simulink library "Control_FuelCell1Motor"  (R2026a)
settings: Solver=VariableStepAuto
undefined symbols (not defined in the file or in its folder): Coefficient, Control
libraries: simulink x4, Damper_Control_Axle2 x2, sl_discontinuities x2, Driveline_Control_Axle2_None x1, slpidlib x1, Spring_Control_Axle2 x1, Steer_Control_Axle2 x1
Description:
  | Component of Simscape Vehicle Templates Library
  | 
  | Copyright 2018-2026 The MathWorks, Inc.
settings Model: Creator=smiller  LastModifiedBy=smiller

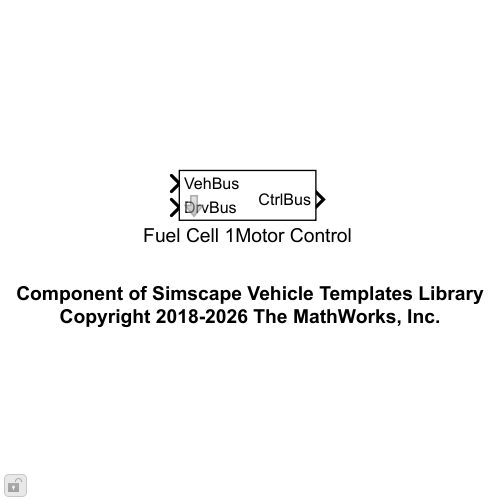
[thumbnail: Simulink's stored preview of the top-level diagram]
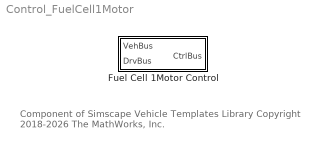
== system Control_FuelCell1Motor ==
  note: Component of Simscape Vehicle Templates Library
      | Copyright 2018-2026 The MathWorks, Inc.
  Fuel Cell 1Motor Control : Subsystem  mask(Control of Fuel Cell Powertrain){ControlFuelCell=Control.FuelCell1Motor, popup_damper_control_A1=Coefficient, popup_damper_control_A2=Coefficient, popup_spring_control_A1=None, popup_spring_control_A2=None}
      mask prompts: ControlFuelCell "Control (structure)"; popup_damper_control_A1 "Damper Control Axle 1"; popup_damper_control_A2 "Damper Control Axle 2"; popup_spring_control_A1 "Spring Control Axle 1"; popup_spring_control_A2 "Spring Control Axle 2"
      mask help: Models control algorithm for fuel cell and regenerative braking of single motor powertrain.
      mask TypeOptions popup_damper_control_A1: Damper Control/popup_damper_control_A1
      mask TypeOptions popup_damper_control_A2: Damper Control/popup_damper_control_A2
      mask TypeOptions popup_spring_control_A1: Spring Control/popup_spring_control_A1
      mask TypeOptions popup_spring_control_A2: Spring Control/popup_spring_control_A2

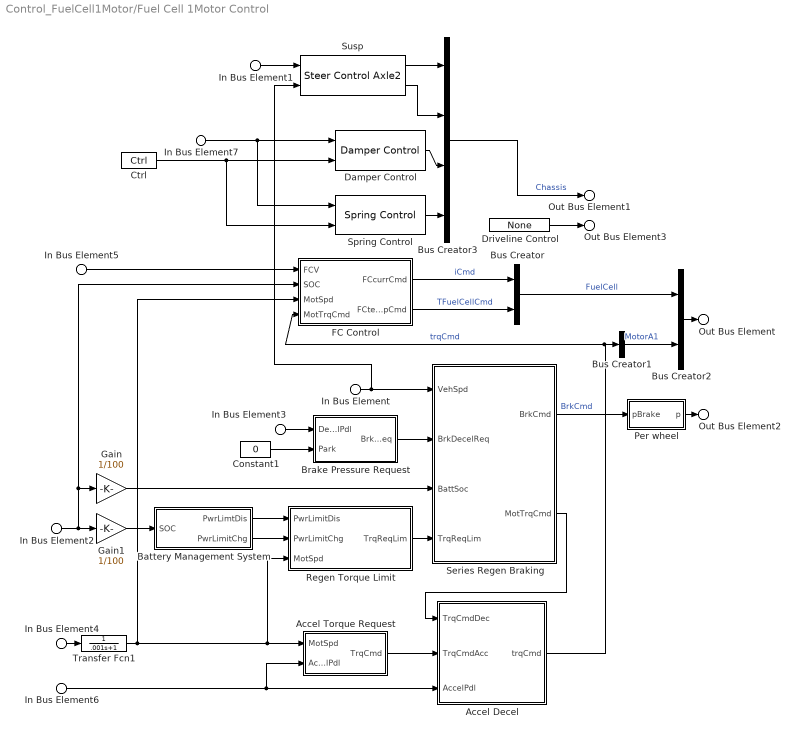
== system Control_FuelCell1Motor/Fuel Cell 1Motor Control ==
  In Bus Element7 : Inport  PortName=VehBus
  In Bus Element : Inport  PortName=VehBus  Element=Chassis.Body.CG.vx
  In Bus Element2 : Inport  PortName=VehBus  Element=Power.Battery.SOC
  In Bus Element5 : Inport  PortName=VehBus  Element=Power.FuelCell.v
  In Bus Element4 : Inport  PortName=VehBus  Element=Power.MotorA1.w
  In Bus Element3 : Inport  Port=2  PortName=DrvBus  Element=rBrakePedal
  In Bus Element6 : Inport  Port=2  PortName=DrvBus  Element=rAccelPedal
  In Bus Element1 : Inport  Port=2  PortName=DrvBus  Element=aSteerWheel
  Accel Decel : Subsystem
  Accel Torque Request : Subsystem
  Battery Management System : Subsystem
  Brake Pressure Request : Subsystem
  Bus Creator : BusCreator  Inputs=2
  Bus Creator1 : BusCreator  Inputs=1
  Bus Creator2 : BusCreator  Inputs=2
  Bus Creator3 : BusCreator  Inputs=4
  Constant1 : Constant  Value=0
  Ctrl : Damper_Control_Axle2/Ctrl  SystemSampleTime=-1  VariantActivationTime=update diagram  EmptyChoice=off  PassThrough=off  PassThroughVariantControl=(default)  EmptyChoiceVariantControl=(default)  AllowFlexibleInterface=on  Latency=0  AutoFrameSizeCalculation=off
  Damper Control : Damper_Control_Axle2/Damper Control  VariantControl=Choice  popup_damper_control_A1=Coefficient  popup_damper_control_A2=Coefficient
  Driveline Control : Driveline_Control_Axle2_None/None  SystemSampleTime=-1  VariantActivationTime=update diagram  EmptyChoice=off  PassThrough=off  PassThroughVariantControl=(default)  EmptyChoiceVariantControl=(default)  AllowFlexibleInterface=on  Latency=0  AutoFrameSizeCalculation=off
  FC Control : Subsystem
  Gain : Gain  Gain=1/100
  Gain1 : Gain  Gain=1/100
  Per wheel : Subsystem
  Regen Torque Limit : Subsystem
  Series Regen Braking : Subsystem  InitFcn=%[~]=autosharedicon('autolibutils',gcb,0);  VariantControl=Variant
  Spring Control : Spring_Control_Axle2/Spring Control  VariantControl=Choice  popup_spring_control_A1=None  popup_gas_spring_A1=Stiff  popup_spring_control_A2=None  popup_gas_spring_A2=Stiff
  Susp : Steer_Control_Axle2/Steer Control Axle2  Steer=ControlFuelCell.Steer
  Transfer Fcn1 : TransferFcn  Denominator=[.001 1]
  Out Bus Element : Outport  PortName=CtrlBus  Element=Power
  Out Bus Element2 : Outport  PortName=CtrlBus  Element=Brakes
  Out Bus Element1 : Outport  PortName=CtrlBus  Element=Chassis
  Out Bus Element3 : Outport  PortName=CtrlBus  Element=Driveline
  wires:
  Accel Decel/1(trqCmd) -> FC Control/4(MotTrqCmd), Bus Creator1/1  "trqCmd"
  In Bus Element6/1 -> Accel Torque Request/2(AccelPdl), Accel Decel/3(AccelPdl)
  Gain1/1 -> Battery Management System/1(SOC)
  In Bus Element4/1 -> Transfer Fcn1/1
  Gain/1 -> Series Regen Braking/3(BattSoc)
  In Bus Element3/1 -> Brake Pressure Request/1(DecelPdl)
  In Bus Element2/1 -> FC Control/2(SOC), Gain/1, Gain1/1
  FC Control/2(FCtempCmd) -> Bus Creator/2  "TFuelCellCmd"
  In Bus Element5/1 -> FC Control/1(FCV)
  FC Control/1(FCcurrCmd) -> Bus Creator/1  "iCmd"
  Bus Creator/1 -> Bus Creator2/1  "FuelCell"
  Bus Creator1/1 -> Bus Creator2/2  "MotorA1"
  Bus Creator2/1 -> Out Bus Element/1
  Transfer Fcn1/1 -> Regen Torque Limit/3(MotSpd), Accel Torque Request/1(MotSpd), FC Control/3(MotSpd)
  Susp/1 -> Bus Creator3/1
  Bus Creator3/1 -> Out Bus Element1/1  "Chassis"
  Susp/2 -> Bus Creator3/2
  Driveline Control/1 -> Out Bus Element3/1
  Series Regen Braking/2(" MotTrqCmd") -> Accel Decel/1(TrqCmdDec)
  Series Regen Braking/1(" BrkCmd") -> Per wheel/1(pBrake)  "BrkCmd"
  Per wheel/1(p) -> Out Bus Element2/1
  Accel Torque Request/1(TrqCmd) -> Accel Decel/2(TrqCmdAcc)
  Regen Torque Limit/1("TrqReqLim ") -> Series Regen Braking/4(TrqReqLim)
  Constant1/1 -> Brake Pressure Request/2(Park)
  Brake Pressure Request/1(BrkDecelReq) -> Series Regen Braking/2(BrkDecelReq)
  Battery Management System/1(PwrLimtDis) -> Regen Torque Limit/1(PwrLimitDis)
  Battery Management System/2(PwrLimitChg) -> Regen Torque Limit/2("PwrLimitChg ")
  In Bus Element1/1 -> Susp/1
  In Bus Element/1 -> Susp/2, Series Regen Braking/1(VehSpd)
  In Bus Element7/1 -> Spring Control/1, Damper Control/1
  Damper Control/1 -> Bus Creator3/3
  Spring Control/1 -> Bus Creator3/4
  Ctrl/1 -> Spring Control/2, Damper Control/2

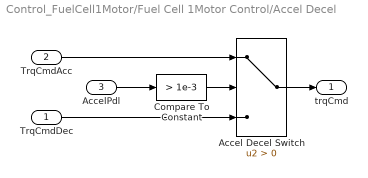
== system Control_FuelCell1Motor/Fuel Cell 1Motor Control/Accel Decel ==
  TrqCmdDec : Inport
  TrqCmdAcc : Inport  Port=2
  AccelPdl : Inport  Port=3
  Accel Decel Switch : Switch  Criteria=u2 > Threshold  SaturateOnIntegerOverflow=off  InputSameDT=off
  Compare To Constant : simulink/Logic and Bit Operations/Compare To Constant  relop=>  const=1e-3  OutDataTypeStr=boolean  ZeroCross=off
  trqCmd : Outport  VectorParamsAs1DForOutWhenUnconnected=off
  wires:
  TrqCmdDec/1 -> Accel Decel Switch/3
  Accel Decel Switch/1 -> trqCmd/1
  TrqCmdAcc/1 -> Accel Decel Switch/1
  AccelPdl/1 -> Compare To Constant/1
  Compare To Constant/1 -> Accel Decel Switch/2

== system Control_FuelCell1Motor/Fuel Cell 1Motor Control/Accel Torque Request ==
  note: Convert Accelerator Pedal Position to Torque Command
      | using Motor Torque Speed Curve
  MotSpd : Inport
  AccelPdl : Inport  Port=2
  MaxMotTrqVsSpd : Lookup_n-D  NumberOfTableDimensions=1  BreakpointsForDimension1=ControlFuelCell.MotorA1.TorqueSpd.w.Value %Mot.w_eff_bp_EV_rear  Table=ControlFuelCell.MotorA1.TorqueSpd.trq.Value % Mot.T_t_EV_rear  ExtrapMethod=Clip  UseLastTableValue=on  InternalRulePriority=Speed  OutDataTypeStr=Inherit: Inherit from 'Table data'  RndMeth=Simplest
  Product1 : Product
  rads_to_rpm : Gain  Gain=30/pi
  TrqCmd : Outport  VectorParamsAs1DForOutWhenUnconnected=off
  wires:
  rads_to_rpm/1 -> MaxMotTrqVsSpd/1
  MotSpd/1 -> rads_to_rpm/1
  AccelPdl/1 -> Product1/1
  MaxMotTrqVsSpd/1 -> Product1/2
  Product1/1 -> TrqCmd/1

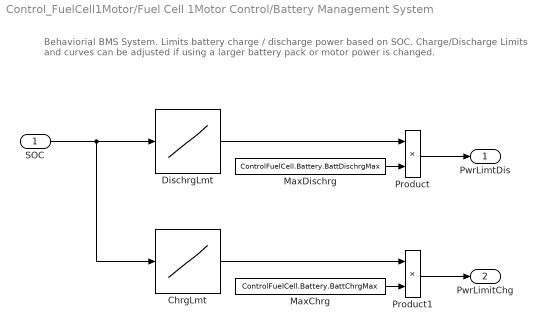
== system Control_FuelCell1Motor/Fuel Cell 1Motor Control/Battery Management System ==
  note: Behaviorial BMS System. Limits battery charge / discharge power based on SOC.
      |
      | Charge/Discharge Limits and curves can be adjusted if using a larger battery pack
      | or motor power is changed.
  SOC : Inport
  ChrgLmt : Lookup_n-D  NumberOfTableDimensions=1  BreakpointsForDimension1=ControlFuelCell.Battery.SOC_bpt  Table=ControlFuelCell.Battery.ChrgLmt_bpt  ExtrapMethod=Clip  UseLastTableValue=on  InternalRulePriority=Speed  RndMeth=Simplest
  DischrgLmt : Lookup_n-D  NumberOfTableDimensions=1  BreakpointsForDimension1=ControlFuelCell.Battery.SOC_bpt  Table=ControlFuelCell.Battery.DischrgLmt_bpt  ExtrapMethod=Clip  UseLastTableValue=on  InternalRulePriority=Speed  RndMeth=Simplest
  MaxChrg : Constant  Value=ControlFuelCell.Battery.BattChrgMax
  MaxDischrg : Constant  Value=ControlFuelCell.Battery.BattDischrgMax
  Product : Product
  Product1 : Product
  PwrLimtDis : Outport  VectorParamsAs1DForOutWhenUnconnected=off
  PwrLimitChg : Outport  Port=2  VectorParamsAs1DForOutWhenUnconnected=off
  wires:
  DischrgLmt/1 -> Product/1
  ChrgLmt/1 -> Product1/1
  Product1/1 -> PwrLimitChg/1
  Product/1 -> PwrLimtDis/1
  MaxDischrg/1 -> Product/2
  MaxChrg/1 -> Product1/2
  SOC/1 -> ChrgLmt/1, DischrgLmt/1

== system Control_FuelCell1Motor/Fuel Cell 1Motor Control/Brake Pressure Request ==
  note: Converts Brake Pedal Position to Deceleration Request
  DecelPdl : Inport
  Park : Inport  Port=2
  Constant1 : Constant
  Switch : Switch  Criteria=u2 > Threshold  ZeroCross=off  SaturateOnIntegerOverflow=off  InputSameDT=off
  BrkDecelReq : Outport  VectorParamsAs1DForOutWhenUnconnected=off
  wires:
  Park/1 -> Switch/2
  Switch/1 -> BrkDecelReq/1
  Constant1/1 -> Switch/1
  DecelPdl/1 -> Switch/3

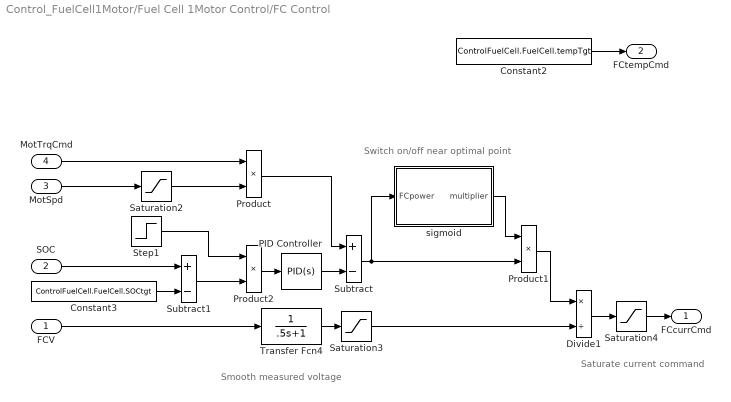
== system Control_FuelCell1Motor/Fuel Cell 1Motor Control/FC Control ==
  note: Switch on/off near optimal point
  note: Smooth measured voltage
  note: Saturate current command
  FCV : Inport
  SOC : Inport  Port=2
  MotSpd : Inport  Port=3
  MotTrqCmd : Inport  Port=4
  Constant2 : Constant  Value=ControlFuelCell.FuelCell.tempTgt
  Constant3 : Constant  Value=ControlFuelCell.FuelCell.SOCtgt
  Divide1 : Product  Inputs=*/
  PID Controller : slpidlib/PID Controller  Controller=PID  Form=Parallel  TimeDomain=Continuous-time  UseExternalTs=off  SampleTime=-1  IntegratorMethod=Forward Euler  FilterMethod=Forward Euler  ControllerParametersSource=internal  P=10000/100  I=0  UseKiTs=off  D=0  UseExternalDerivativeSource=off  N=100  UseFilter=on  TunerSelectOption=Transfer Function Based (PID Tuner App)  ZeroCross=off  InitialConditionSource=internal  InitialConditionForIntegrator=0  InitialConditionForFilter=0  DifferentiatorICPrevScaledInput=0  ExternalReset=none  TrackingMode=off  Kt=1  LimitOutput=off  SatLimitsSource=internal  UpperSaturationLimit=inf  LowerSaturationLimit=-inf  LinearizeAsGain=on  AntiWindupMode=none  Kb=1  LimitIntegrator=off  UpperIntegratorSaturationLimit=inf  LowerIntegratorSaturationLimit=-inf  POutMin=[]  POutMax=[]  IOutMin=[]  IOutMax=[]  DOutMin=[]  DOutMax=[]  NOutMin=[]  NOutMax=[]  SumOutMin=[]  SumOutMax=[]  SaturationOutMin=[]  SaturationOutMax=[]  PParamMin=[]  PParamMax=[]  IParamMin=[]  IParamMax=[]  DParamMin=[]  DParamMax=[]  NParamMin=[]  NParamMax=[]  KbParamMin=[]  KbParamMax=[]  KtParamMin=[]  KtParamMax=[]  KbOutMin=[]  KbOutMax=[]  KtOutMin=[]  KtOutMax=[]  IntegratorOutMin=[]  IntegratorOutMax=[]  FilterOutMin=[]  FilterOutMax=[]  SumI1OutMin=[]  SumI1OutMax=[]  SumI2OutMin=[]  SumI2OutMax=[]  SumI3OutMin=[]  SumI3OutMax=[]  SumI4OutMin=[]  SumI4OutMax=[]  SumDOutMin=[]  SumDOutMax=[]  DifferentiatorOutMin=[]  DifferentiatorOutMax=[]  FilterDiffOutCoefMin=[]  FilterDiffOutCoefMax=[]  ReciprocalOutMin=[]  ReciprocalOutMax=[]  SumDenOutMin=[]  SumDenOutMax=[]  SumNumOutMin=[]  SumNumOutMax=[]  DivideOutMin=[]  DivideOutMax=[]  UdiffTsProdOutMin=[]  UdiffTsProdOutMax=[]  NTsProdOutMin=[]  NTsProdOutMax=[]  UintegralTsProdOutMin=[]  UintegralTsProdOutMax=[]  UngainTsProdOutMin=[]  UngainTsProdOutMax=[]  ClampingZeroOutDataTypeStr=Inherit: Inherit via back propagation  ClampingZeroOutMin=[]  ClampingZeroOutMax=[]  FilterDenConstantOutDataTypeStr=Inherit: Inherit via back propagation  FilterDenConstantOutMin=[]  FilterDenConstantOutMax=[]  PCopyOutDataTypeStr=Inherit: Inherit via back propagation  PCopyOutMin=[]  PCopyOutMax=[]  NCopyOutDataTypeStr=Inherit: Inherit via back propagation  NCopyOutMin=[]  NCopyOutMax=[]  IntegratorContinuousStateAttributes=''  IntegratorStateMustResolveToSignalObject=off  IntegratorRTWStateStorageClass=Auto  FilterContinuousStateAttributes=''  FilterStateMustResolveToSignalObject=off  FilterRTWStateStorageClass=Auto  ParallelPVariant=InternalParameters  IdealPVariant=Disabled  IVariant=InternalParameters  DVariant=InternalParameters  IntegratorVariant=Continuous  SatVariant=Disabled  AWVariant=Passthrough  PCopyVariant=Disabled  TRVariant=Disabled  FdbkBlocksVariant=Forward  IdealPFdbkVariant=Disabled  SatFdbkVariant=Disabled  DerivativeFilterVariant=ContFilter  NVariant=InternalParameters  NCopyVariant=Disabled  FilterICVariant=InternalICsFilter  IntegratorICVariant=InternalICs  ExternalResetVariant=Disabled  TRSumVariant=Passthrough  SumFdbkVariant=Disabled  SumVariant=Sum_PID  TsampFilterVariant=InternalTs  TsampNgainVariant=Passthrough  TsampIntegralVariant=Disabled_SignalSpec  ExternalSaturationOutDataTypeStr=Inherit: Same as second input  DerivativeSourceVariant=ErrorSignal  PreIntVariant=InternalPreInt
  Product : Product
  Product1 : Product
  Product2 : Product
  Saturation2 : Saturate  UpperLimit=inf  LowerLimit=1  ZeroCross=off
  Saturation3 : Saturate  UpperLimit=inf  LowerLimit=200  ZeroCross=off
  Saturation4 : Saturate  UpperLimit=350  LowerLimit=0  ZeroCross=off
  Step1 : Step  SampleTime=0
  Subtract : Sum  Inputs=+-
  Subtract1 : Sum  Inputs=+-
  Transfer Fcn4 : TransferFcn  Denominator=[.5 1]
  sigmoid : Subsystem
  FCcurrCmd : Outport
  FCtempCmd : Outport  Port=2
  wires:
  PID Controller/1 -> Subtract/2
  Transfer Fcn4/1 -> Saturation3/1
  Saturation3/1 -> Divide1/2
  SOC/1 -> Subtract1/1
  Step1/1 -> Product2/1
  Constant3/1 -> Subtract1/2
  Saturation4/1 -> FCcurrCmd/1
  FCV/1 -> Transfer Fcn4/1
  Divide1/1 -> Saturation4/1
  Saturation2/1 -> Product/2
  MotTrqCmd/1 -> Product/1
  Subtract1/1 -> Product2/2
  MotSpd/1 -> Saturation2/1
  Constant2/1 -> FCtempCmd/1
  Product2/1 -> PID Controller/1
  Product/1 -> Subtract/1
  Product1/1 -> Divide1/1
  sigmoid/1(multiplier) -> Product1/1
  Subtract/1 -> Product1/2, sigmoid/1(FCpower)

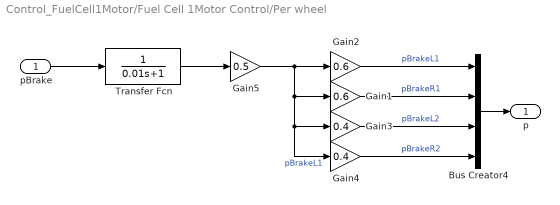
== system Control_FuelCell1Motor/Fuel Cell 1Motor Control/Per wheel ==
  pBrake : Inport
  Bus Creator4 : BusCreator  Inputs=4
  Gain1 : Gain  Gain=0.6
  Gain2 : Gain  Gain=0.6
  Gain3 : Gain  Gain=0.4
  Gain4 : Gain  Gain=0.4
  Gain5 : Gain  Gain=0.5
  Transfer Fcn : TransferFcn  Denominator=[0.01 1]
  p : Outport  VectorParamsAs1DForOutWhenUnconnected=off
  wires:
  Gain4/1 -> Bus Creator4/4  "pBrakeR2"
  Gain3/1 -> Bus Creator4/3  "pBrakeL2"
  Gain1/1 -> Bus Creator4/2  "pBrakeR1"
  Bus Creator4/1 -> p/1
  pBrake/1 -> Transfer Fcn/1
  Gain2/1 -> Bus Creator4/1  "pBrakeL1"
  Gain5/1 -> Gain2/1, Gain1/1, Gain3/1, Gain4/1  "pBrakeL1"
  Transfer Fcn/1 -> Gain5/1

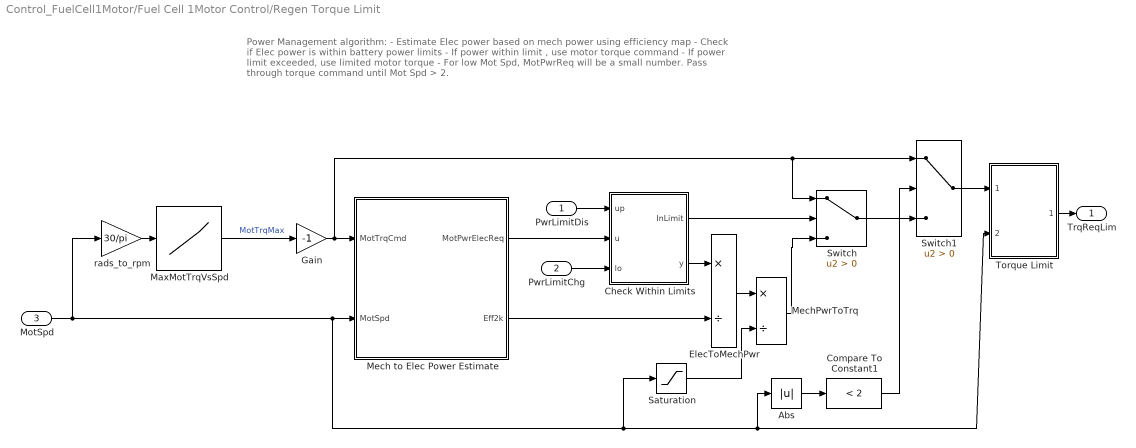
== system Control_FuelCell1Motor/Fuel Cell 1Motor Control/Regen Torque Limit ==
  note: Power Management algorithm:
      | - Estimate Elec power based on mech power using efficiency map
      | - Check if Elec power is within battery power limits
      | - If power within limit , use motor torque command
      | - If power limit exceeded, use limited motor torque
      | - For low Mot Spd, MotPwrReq will be a small number.  Pass through torque command until Mot Spd > 2.
  PwrLimitDis : Inport
  "PwrLimitChg " : Inport  Port=2
  MotSpd : Inport  Port=3
  Abs : Abs  ZeroCross=off  SaturateOnIntegerOverflow=off
  Check Within Limits : Subsystem
  Compare To Constant1 : simulink/Logic and Bit Operations/Compare To Constant  relop=<  const=2  OutDataTypeStr=boolean  ZeroCross=off
  ElecToMechPwr : Product  Inputs=*/
  Gain : Gain  Gain=-1
  MaxMotTrqVsSpd : Lookup_n-D  NumberOfTableDimensions=1  BreakpointsForDimension1=ControlFuelCell.MotorA1.TorqueSpd.w.Value  Table=ControlFuelCell.MotorA1.TorqueSpd.trq.Value  ExtrapMethod=Clip  UseLastTableValue=on  InternalRulePriority=Speed  OutDataTypeStr=Inherit: Inherit from 'Table data'  RndMeth=Simplest
  Mech to Elec Power Estimate : Subsystem
  MechPwrToTrq : Product  Inputs=*/
  Saturation : Saturate  UpperLimit=inf  LowerLimit=2
  Switch : Switch  Criteria=u2 > Threshold  ZeroCross=off  SaturateOnIntegerOverflow=off  InputSameDT=off
  Switch1 : Switch  Criteria=u2 > Threshold  ZeroCross=off  SaturateOnIntegerOverflow=off  InputSameDT=off
  Torque Limit : Subsystem
  rads_to_rpm : Gain  Gain=30/pi
  "TrqReqLim " : Outport  VectorParamsAs1DForOutWhenUnconnected=off
  wires:
  Switch1/1 -> Torque Limit/1(MotTrq)
  Torque Limit/1(MotReqCmd) -> "TrqReqLim "/1
  Mech to Elec Power Estimate/2(Eff2k) -> ElecToMechPwr/2
  PwrLimitDis/1 -> Check Within Limits/1(up)
  "PwrLimitChg "/1 -> Check Within Limits/3(lo)
  Gain/1 -> Mech to Elec Power Estimate/1(MotTrqCmd), Switch1/1, Switch/1
  Check Within Limits/1(InLimit) -> Switch/2
  Check Within Limits/2(y) -> ElecToMechPwr/1
  Mech to Elec Power Estimate/1(MotPwrElecReq) -> Check Within Limits/2(u)
  Switch/1 -> Switch1/3
  Abs/1 -> Compare To Constant1/1
  Compare To Constant1/1 -> Switch1/2
  Saturation/1 -> MechPwrToTrq/2
  MechPwrToTrq/1 -> Switch/3
  ElecToMechPwr/1 -> MechPwrToTrq/1
  rads_to_rpm/1 -> MaxMotTrqVsSpd/1
  MaxMotTrqVsSpd/1 -> Gain/1  "MotTrqMax"
  MotSpd/1 -> Torque Limit/2(MotSpd), Abs/1, Saturation/1, Mech to Elec Power Estimate/2(MotSpd), rads_to_rpm/1

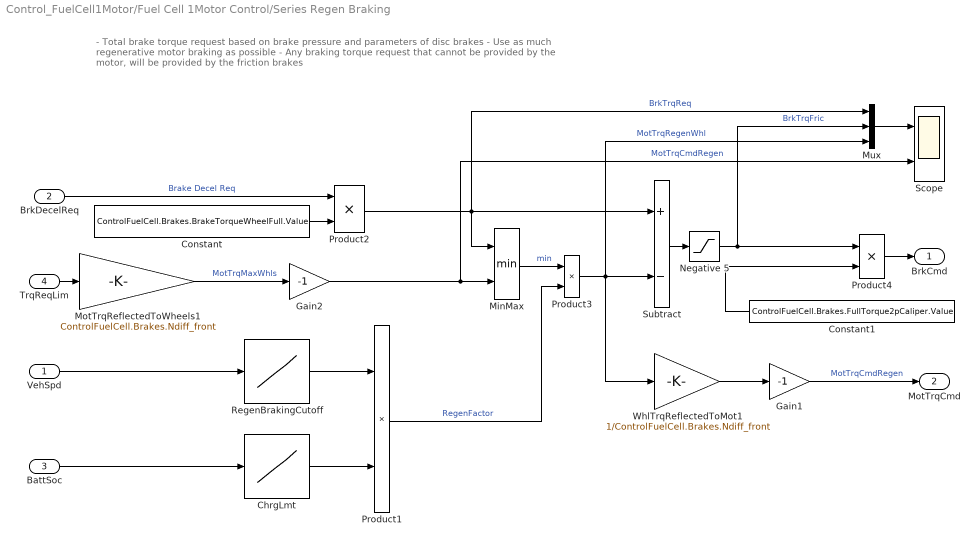
== system Control_FuelCell1Motor/Fuel Cell 1Motor Control/Series Regen Braking ==
  note: - Total brake torque request based on brake pressure and parameters of disc brakes
      | - Use as much regenerative motor braking as possible
      | - Any braking torque request that cannot be provided by the motor, will be provided by the friction brakes
  VehSpd : Inport
  BrkDecelReq : Inport  Port=2
  BattSoc : Inport  Port=3
  TrqReqLim : Inport  Port=4
  ChrgLmt : Lookup_n-D  NumberOfTableDimensions=1  BreakpointsForDimension1=ControlFuelCell.Battery.SOC_bpt  Table=ControlFuelCell.Battery.ChrgLmt_bpt  ExtrapMethod=Clip  UseLastTableValue=on  InternalRulePriority=Speed  RndMeth=Simplest
  Constant : Constant  Value=ControlFuelCell.Brakes.BrakeTorqueWheelFull.Value
  Constant1 : Constant  Value=ControlFuelCell.Brakes.FullTorque2pCaliper.Value
  Gain1 : Gain  Gain=-1
  Gain2 : Gain  Gain=-1
  MinMax : MinMax  Inputs=2
  MotTrqReflectedToWheels1 : Gain  Gain=ControlFuelCell.Brakes.Ndiff_front
  Mux : Mux  Inputs=3
  Negative 5 : Saturate  UpperLimit=inf  LowerLimit=0  ZeroCross=off
  Product1 : Product
  Product2 : Product
  Product3 : Product
  Product4 : Product  Inputs=**
  RegenBrakingCutoff : Lookup_n-D  NumberOfTableDimensions=1  BreakpointsForDimension1=ControlFuelCell.Power.RegenBrkSpd_bpt  Table=ControlFuelCell.Power.RegenBrkCutOff  ExtrapMethod=Clip  UseLastTableValue=on  InternalRulePriority=Speed  RndMeth=Simplest
  Scope : Scope  NumInputPorts=2
      settings: ActiveDisplayYMinimum=-294.72625  ActiveDisplayYMaximum=2652.53625
  Subtract : Sum  Inputs=+-
  WhlTrqReflectedToMot1 : Gain  Gain=1/ControlFuelCell.Brakes.Ndiff_front
  " BrkCmd" : Outport  VectorParamsAs1DForOutWhenUnconnected=off
  " MotTrqCmd" : Outport  Port=2  VectorParamsAs1DForOutWhenUnconnected=off
  wires:
  Product4/1 -> " BrkCmd"/1
  Negative 5/1 -> Product4/1, Mux/2  "BrkTrqFric"
  BattSoc/1 -> ChrgLmt/1
  Subtract/1 -> Negative 5/1
  Product1/1 -> Product3/2  "RegenFactor"
  RegenBrakingCutoff/1 -> Product1/1
  VehSpd/1 -> RegenBrakingCutoff/1
  ChrgLmt/1 -> Product1/2
  MinMax/1 -> Product3/1  "min"
  Product2/1 -> MinMax/1, Subtract/1, Mux/1  "BrkTrqReq"
  BrkDecelReq/1 -> Product2/1  "Brake Decel Req"
  Constant/1 -> Product2/2
  Constant1/1 -> Product4/2
  Product3/1 -> WhlTrqReflectedToMot1/1, Subtract/2, Mux/3  "MotTrqRegenWhl"
  Mux/1 -> Scope/1
  TrqReqLim/1 -> MotTrqReflectedToWheels1/1
  WhlTrqReflectedToMot1/1 -> Gain1/1
  Gain1/1 -> " MotTrqCmd"/1  "MotTrqCmdRegen"
  Gain2/1 -> MinMax/2, Scope/2  "MotTrqCmdRegen"
  MotTrqReflectedToWheels1/1 -> Gain2/1  "MotTrqMaxWhls"

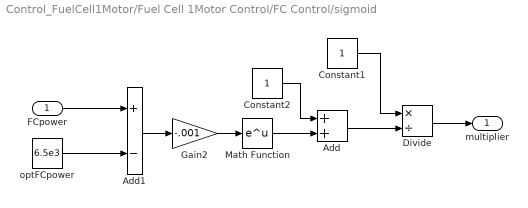
== system Control_FuelCell1Motor/Fuel Cell 1Motor Control/FC Control/sigmoid ==
  FCpower : Inport
  Add : Sum
  Add1 : Sum  Inputs=+-
  Constant1 : Constant
  Constant2 : Constant
  Divide : Product  Inputs=*/
  Gain2 : Gain  Gain=-.001
  Math Function : Math  SignedPower=on
  optFCpower : Constant  Value=6.5e3
  multiplier : Outport
  wires:
  Add1/1 -> Gain2/1
  Divide/1 -> multiplier/1
  Math Function/1 -> Add/2
  Add/1 -> Divide/2
  optFCpower/1 -> Add1/2
  Constant2/1 -> Add/1
  FCpower/1 -> Add1/1
  Gain2/1 -> Math Function/1
  Constant1/1 -> Divide/1

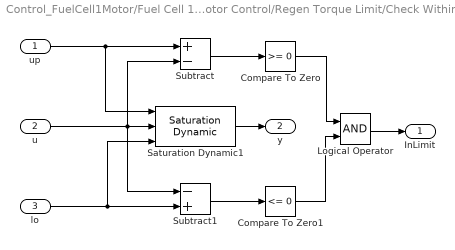
== system Control_FuelCell1Motor/Fuel Cell 1Motor Control/Regen Torque Limit/Check Within Limits ==
  up : Inport
  u : Inport  Port=2
  lo : Inport  Port=3
  Compare To Zero : simulink/Logic and Bit Operations/Compare To Zero  relop=>=  OutDataTypeStr=boolean
  Compare To Zero1 : simulink/Logic and Bit Operations/Compare To Zero  relop=<=  OutDataTypeStr=boolean
  Logical Operator : Logic  AllPortsSameDT=off  OutDataTypeStr=boolean
  Saturation Dynamic1 : sl_discontinuities/Saturation Dynamic  OutMin=[]  OutMax=[]  OutDataTypeStr=Inherit: Same as second input  OutDataType=fixdt(1, 16)  OutScaling=2^-10  DoSatur=off
  Subtract : Sum  Inputs=+-
  Subtract1 : Sum  Inputs=-+
  InLimit : Outport  SampleTime=0  VectorParamsAs1DForOutWhenUnconnected=off
  y : Outport  Port=2  VectorParamsAs1DForOutWhenUnconnected=off
  wires:
  Logical Operator/1 -> InLimit/1
  Compare To Zero1/1 -> Logical Operator/2
  Compare To Zero/1 -> Logical Operator/1
  Subtract1/1 -> Compare To Zero1/1
  Subtract/1 -> Compare To Zero/1
  u/1 -> Saturation Dynamic1/2, Subtract/2, Subtract1/1
  up/1 -> Saturation Dynamic1/1, Subtract/1
  lo/1 -> Saturation Dynamic1/3, Subtract1/2
  Saturation Dynamic1/1 -> y/1

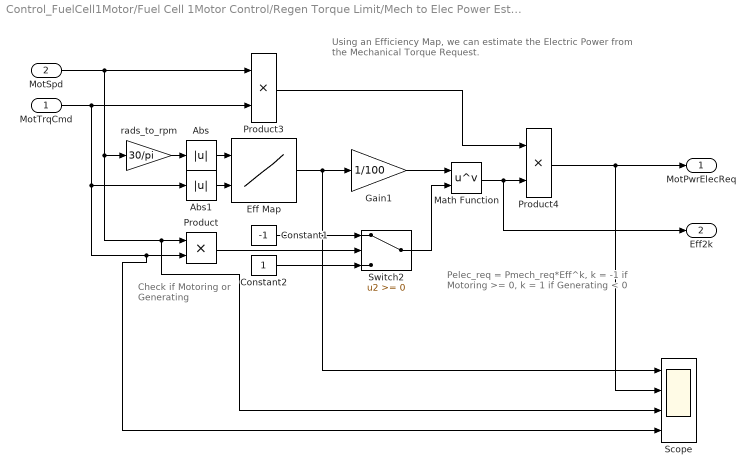
== system Control_FuelCell1Motor/Fuel Cell 1Motor Control/Regen Torque Limit/Mech to Elec Power Estimate ==
  note: Pelec_req = Pmech_req*Eff^k,
      | k = -1 if Motoring >= 0,
      | k = 1 if Generating < 0
  note: Using an Efficiency Map, we can estimate the
      | Electric Power from the Mechanical  Torque Request.
  note: Check if Motoring
      | or Generating
  MotTrqCmd : Inport
  MotSpd : Inport  Port=2
  Abs : Abs  ZeroCross=off  SaturateOnIntegerOverflow=off
  Abs1 : Abs  ZeroCross=off  SaturateOnIntegerOverflow=off
  Constant1 : Constant  Value=-1  SampleTime=0
  Constant2 : Constant  SampleTime=0
  Eff Map : Lookup_n-D  BreakpointsForDimension1=ControlFuelCell.MotorA1.LossTable.w.Value  BreakpointsForDimension2=ControlFuelCell.MotorA1.LossTable.trq.Value  Table=ControlFuelCell.MotorA1.LossTable.efficiency.Value  ExtrapMethod=Clip  UseLastTableValue=on  InternalRulePriority=Speed  OutDataTypeStr=Inherit: Inherit from 'Table data'  RndMeth=Simplest
      settings: InputPortMap=u0,u1
  Gain1 : Gain  Gain=1/100
  Math Function : Math  Operator=pow  SignedPower=on  OutputSignalType=real
  Product : Product
  Product3 : Product
  Product4 : Product
  Scope : Scope  NumInputPorts=4
      settings: ActiveDisplayYMinimum=84.125  ActiveDisplayYMaximum=92.875  DataLoggingVariableName=ScopeData2
  Switch2 : Switch  ZeroCross=off  SaturateOnIntegerOverflow=off  InputSameDT=off
  rads_to_rpm : Gain  Gain=30/pi
  MotPwrElecReq : Outport  VectorParamsAs1DForOutWhenUnconnected=off
  Eff2k : Outport  Port=2  VectorParamsAs1DForOutWhenUnconnected=off
  wires:
  MotTrqCmd/1 -> Abs1/1, Scope/4, Product/2, Product3/2
  MotSpd/1 -> rads_to_rpm/1, Scope/3, Product/1, Product3/1
  Product/1 -> Switch2/2
  rads_to_rpm/1 -> Abs/1
  Abs1/1 -> Eff Map/2
  Product4/1 -> Scope/2, MotPwrElecReq/1
  Math Function/1 -> Product4/2, Eff2k/1
  Gain1/1 -> Math Function/1
  Abs/1 -> Eff Map/1
  Eff Map/1 -> Scope/1, Gain1/1
  Constant2/1 -> Switch2/3
  Constant1/1 -> Switch2/1
  Switch2/1 -> Math Function/2
  Product3/1 -> Product4/1

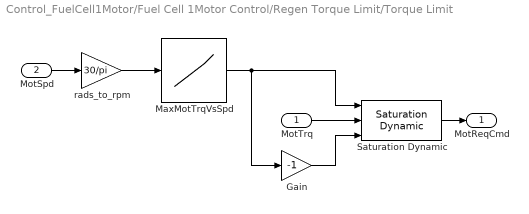
== system Control_FuelCell1Motor/Fuel Cell 1Motor Control/Regen Torque Limit/Torque Limit ==
  MotTrq : Inport
  MotSpd : Inport  Port=2
  Gain : Gain  Gain=-1
  MaxMotTrqVsSpd : Lookup_n-D  NumberOfTableDimensions=1  BreakpointsForDimension1=ControlFuelCell.MotorA1.TorqueSpd.w.Value  Table=ControlFuelCell.MotorA1.TorqueSpd.trq.Value  ExtrapMethod=Clip  UseLastTableValue=on  InternalRulePriority=Speed  OutDataTypeStr=Inherit: Inherit from 'Table data'  RndMeth=Simplest
  Saturation Dynamic : sl_discontinuities/Saturation Dynamic  OutMin=[]  OutMax=[]  OutDataTypeStr=Inherit: Same as second input  OutDataType=fixdt(1, 16)  OutScaling=2^-10  DoSatur=off
  rads_to_rpm : Gain  Gain=30/pi
  MotReqCmd : Outport  VectorParamsAs1DForOutWhenUnconnected=off
  wires:
  Saturation Dynamic/1 -> MotReqCmd/1
  Gain/1 -> Saturation Dynamic/3
  rads_to_rpm/1 -> MaxMotTrqVsSpd/1
  MaxMotTrqVsSpd/1 -> Saturation Dynamic/1, Gain/1
  MotSpd/1 -> rads_to_rpm/1
  MotTrq/1 -> Saturation Dynamic/2
